simulink model "DinamicaCinematicaControleAtitude"  (R2024a)
settings: Solver=FixedStepAuto  StartTime=0.0  StopTime=tf  FixedStep=step_modelo  RelTol=1e-3
undefined symbols (not defined in the file or in its folder): giro, giro_bias, giro_ruido, Ixx, Iyy, Izz, omega1_rel_ini, omega2_rel_ini, omega3_rel_ini, phi_i, psi_i, theta_i
libraries: dspsrcs4 x3, matrix_library x2, aerolibutil x1
settings Model: Creator=rodri  LastModifiedBy=rodri
settings DataIOCC: SaveOutput=off  SaveTime=off
settings RTWCC: GPUComputeCapability=3.5

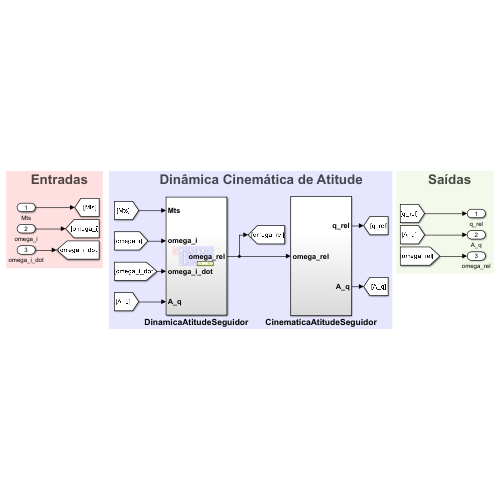
[thumbnail: Simulink's stored preview of the top-level diagram]
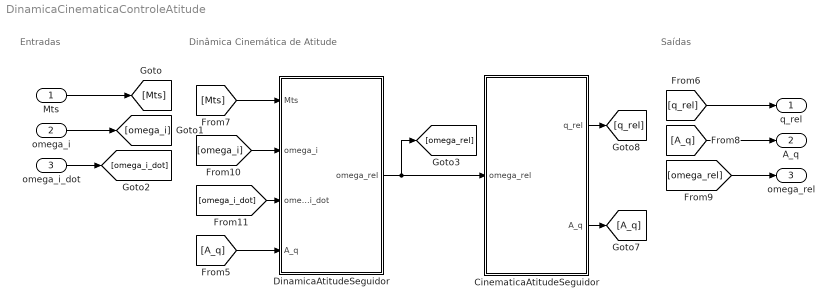
== system DinamicaCinematicaControleAtitude ==
  note: Dinâmica Cinemática de Atitude
  note: Entradas
  note: Saídas
  Mts : Inport  OutDataTypeStr=double  PortDimensions=[3,1]
  omega_i : Inport  Port=2  OutDataTypeStr=double
  omega_i_dot : Inport  Port=3  OutDataTypeStr=double  PortDimensions=[3,1]
  CinematicaAtitudeSeguidor : Subsystem
  DinamicaAtitudeSeguidor : Subsystem
  q_rel : Outport
  A_q : Outport  Port=2  PortDimensions=[3,3]
  omega_rel : Outport  Port=3
  wires:
  DinamicaAtitudeSeguidor/1(omega_rel) -> [omega_rel], CinematicaAtitudeSeguidor/1(omega_rel)
  CinematicaAtitudeSeguidor/2(A_q) -> [A_q]
  CinematicaAtitudeSeguidor/1(q_rel) -> [q_rel]
  omega_i/1 -> [omega_i]
  omega_i_dot/1 -> [omega_i_dot]
  [A_q] -> DinamicaAtitudeSeguidor/4(A_q)
  [Mts] -> DinamicaAtitudeSeguidor/1(Mts)
  [omega_i] -> DinamicaAtitudeSeguidor/2(omega_i)
  [omega_i_dot] -> DinamicaAtitudeSeguidor/3(omega_i_dot)
  [q_rel] -> q_rel/1
  [A_q] -> A_q/1
  [omega_rel] -> omega_rel/1
  Mts/1 -> [Mts]

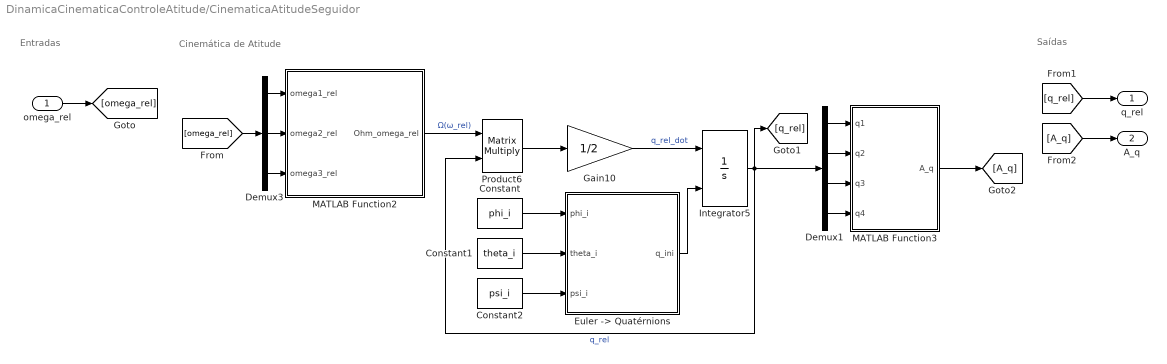
== system DinamicaCinematicaControleAtitude/CinematicaAtitudeSeguidor ==
  note: Cinemática de Atitude
  note: Entradas
  note: Saídas
  omega_rel : Inport
  Constant : Constant  Value=phi_i  SampleTime=-1
  Constant1 : Constant  Value=theta_i  SampleTime=-1
  Constant2 : Constant  Value=psi_i  SampleTime=-1
  Demux1 : Demux
  Demux3 : Demux  Outputs=3
  "Euler -> Quatérnions" : MATLAB Function  TreatAsAtomicUnit=on
  Gain10 : Gain  Gain=1/2
  Integrator5 : Integrator  InitialConditionSource=external  InitialCondition=[1; 0; 0; 0]
  MATLAB Function2 : MATLAB Function  TreatAsAtomicUnit=on
  MATLAB Function3 : MATLAB Function  TreatAsAtomicUnit=on
  Product6 : Product  Multiplication=Matrix(*)
  q_rel : Outport
  A_q : Outport  Port=2  PortDimensions=[3,3]
  wires:
  "Euler -> Quatérnions"/1(q_ini) -> Integrator5/2
  Demux1/2 -> MATLAB Function3/2(q2)
  Demux3/1 -> MATLAB Function2/1(omega1_rel)
  MATLAB Function2/1(Ohm_omega_rel) -> Product6/1  "Ω(ω_rel)"
  Demux1/4 -> MATLAB Function3/4(q4)
  Demux3/3 -> MATLAB Function2/3(omega3_rel)
  Demux3/2 -> MATLAB Function2/2(omega2_rel)
  Integrator5/1 -> Product6/2, Demux1/1, [q_rel]  "q_rel"
  Demux1/3 -> MATLAB Function3/3(q3)
  Gain10/1 -> Integrator5/1  "q_rel_dot"
  Demux1/1 -> MATLAB Function3/1(q1)
  Product6/1 -> Gain10/1
  [omega_rel] -> Demux3/1
  omega_rel/1 -> [omega_rel]
  [q_rel] -> q_rel/1
  [A_q] -> A_q/1
  MATLAB Function3/1(A_q) -> [A_q]
  Constant/1 -> "Euler -> Quatérnions"/1(phi_i)
  Constant1/1 -> "Euler -> Quatérnions"/2(theta_i)
  Constant2/1 -> "Euler -> Quatérnions"/3(psi_i)

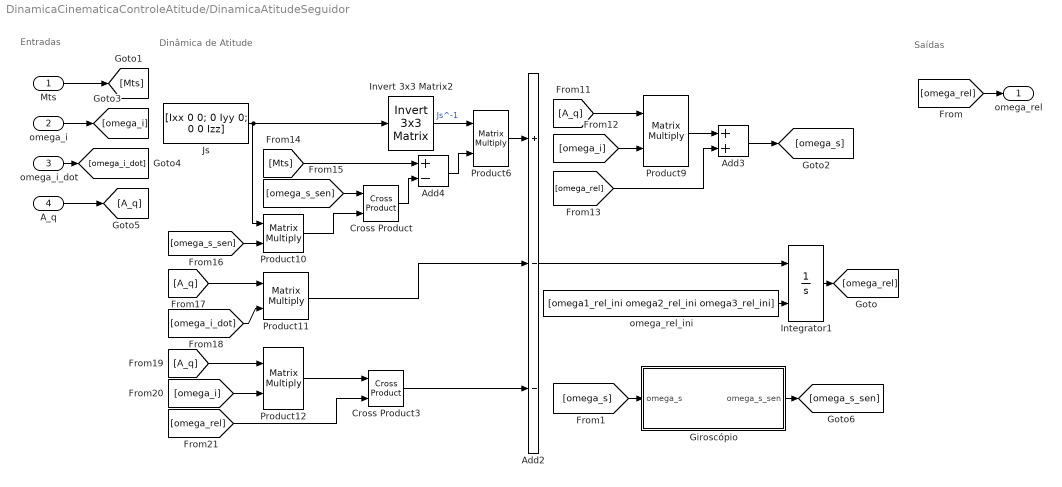
== system DinamicaCinematicaControleAtitude/DinamicaAtitudeSeguidor ==
  note: Dinâmica de Atitude
  note: Saídas
  note: Entradas
  Mts : Inport
  omega_i : Inport  Port=2
  omega_i_dot : Inport  Port=3
  A_q : Inport  Port=4
  Add2 : Sum  Inputs=+--
  Add3 : Sum
  Add4 : Sum  Inputs=+-
  Cross Product : matrix_library/Cross Product
  Cross Product3 : matrix_library/Cross Product
  Giroscópio : Subsystem
  Integrator1 : Integrator  InitialConditionSource=external  InitialCondition=[0; 0; 0]
  Invert 3x3 Matrix2 : aerolibutil/Invert  3x3 Matrix
  Js : Constant  Value=[Ixx 0 0; 0 Iyy 0; 0 0 Izz]
  Product{6,9..12} (5 alike) : Product  Multiplication=Matrix(*)
  omega_rel_ini : Constant  Value=[omega1_rel_ini omega2_rel_ini omega3_rel_ini]
  omega_rel : Outport
  wires:
  Integrator1/1 -> [omega_rel]
  Add2/1 -> Integrator1/1
  Invert 3x3 Matrix2/1 -> Product6/1  "Js^-1"
  omega_rel_ini/1 -> Integrator1/2
  [A_q] -> Product9/1
  [omega_i] -> Product9/2
  Product9/1 -> Add3/1
  [omega_rel] -> Add3/2
  Add3/1 -> [omega_s]
  [Mts] -> Add4/1
  Cross Product/1 -> Add4/2
  [omega_s_sen] -> Cross Product/1
  Js/1 -> Product10/1, Invert 3x3 Matrix2/1
  [omega_s_sen] -> Product10/2
  Product10/1 -> Cross Product/2
  Add4/1 -> Product6/2
  Product6/1 -> Add2/1
  [A_q] -> Product11/1
  [omega_i_dot] -> Product11/2
  Product11/1 -> Add2/2
  [A_q] -> Product12/1
  [omega_i] -> Product12/2
  Product12/1 -> Cross Product3/1
  [omega_rel] -> Cross Product3/2
  Cross Product3/1 -> Add2/3
  omega_i/1 -> [omega_i]
  A_q/1 -> [A_q]
  [omega_rel] -> omega_rel/1
  Mts/1 -> [Mts]
  omega_i_dot/1 -> [omega_i_dot]
  [omega_s] -> Giroscópio/1(omega_s)
  Giroscópio/1(omega_s_sen) -> [omega_s_sen]

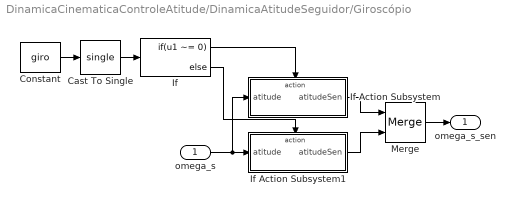
== system DinamicaCinematicaControleAtitude/DinamicaAtitudeSeguidor/Giroscópio ==
  omega_s : Inport
  Cast To Single : DataTypeConversion  OutDataTypeStr=single  SaturateOnIntegerOverflow=off  RndMeth=Floor
  Constant : Constant  Value=giro
  If : If  IfExpression=u1 ~= 0
  If Action Subsystem : Subsystem  TreatAsAtomicUnit=on
  If Action Subsystem1 : Subsystem  TreatAsAtomicUnit=on
  Merge : Merge
  omega_s_sen : Outport
  wires:
  Cast To Single/1 -> If/1
  If/2 -> If Action Subsystem1/Action
  If Action Subsystem/1(atitudeSen) -> Merge/1
  If/1 -> If Action Subsystem/Action
  Merge/1 -> omega_s_sen/1
  Constant/1 -> Cast To Single/1
  If Action Subsystem1/1(atitudeSen) -> Merge/2
  omega_s/1 -> If Action Subsystem/1(atitude), If Action Subsystem1/1(atitude)

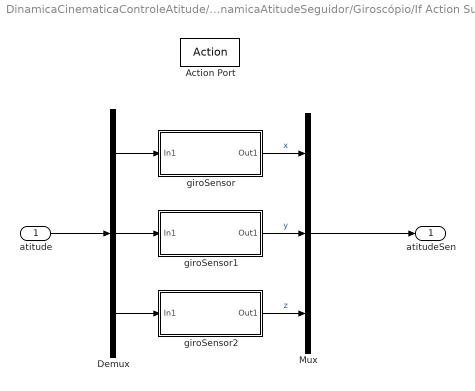
== system DinamicaCinematicaControleAtitude/DinamicaAtitudeSeguidor/Giroscópio/If Action Subsystem ==
  atitude : Inport
  Action Port : ActionPort  ActionPortLabel=if(u1 ~= 0)
  Demux : Demux  Outputs=3
  Mux : Mux  Inputs=3
  giroSensor : Subsystem
  giroSensor1 : Subsystem
  giroSensor2 : Subsystem
  atitudeSen : Outport
  wires:
  Demux/3 -> giroSensor2/1(In1)
  Demux/2 -> giroSensor1/1(In1)
  Demux/1 -> giroSensor/1(In1)
  atitude/1 -> Demux/1
  giroSensor/1(Out1) -> Mux/1  "x"
  giroSensor1/1(Out1) -> Mux/2  "y"
  giroSensor2/1(Out1) -> Mux/3  "z"
  Mux/1 -> atitudeSen/1

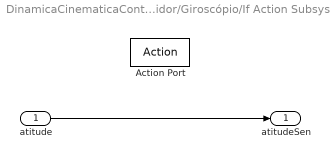
== system DinamicaCinematicaControleAtitude/DinamicaAtitudeSeguidor/Giroscópio/If Action Subsystem1 ==
  atitude : Inport
  Action Port : ActionPort  ActionPortLabel=else
  atitudeSen : Outport
  wires:
  atitude/1 -> atitudeSen/1

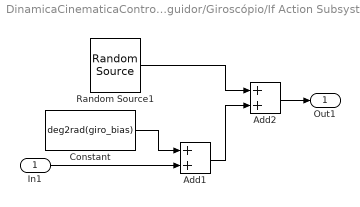
== system DinamicaCinematicaControleAtitude/DinamicaAtitudeSeguidor/Giroscópio/If Action Subsystem/giroSensor ==
  In1 : Inport
  Add1 : Sum
  Add2 : Sum
  Constant : Constant  Value=deg2rad(giro_bias)
  Random Source1 : dspsrcs4/Random Source  SrcType=Uniform  MinVal=-deg2rad(giro_ruido)  MaxVal=deg2rad(giro_ruido)  MeanVal=0  VarVal=1  RepMode=Not repeatable  rawSeed=1  IsInherit=off  SampTime=step_modelo  SampFrame=1  OutComplex=Real  DataType=double  SimulateUsing=Code generation
  Out1 : Outport
  wires:
  Random Source1/1 -> Add2/1
  In1/1 -> Add1/2
  Constant/1 -> Add1/1
  Add1/1 -> Add2/2
  Add2/1 -> Out1/1

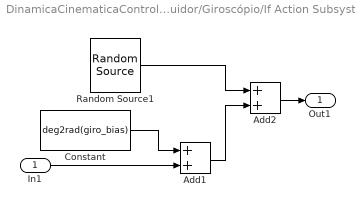
== system DinamicaCinematicaControleAtitude/DinamicaAtitudeSeguidor/Giroscópio/If Action Subsystem/giroSensor1 ==
  In1 : Inport
  Add1 : Sum
  Add2 : Sum
  Constant : Constant  Value=deg2rad(giro_bias)
  Random Source1 : dspsrcs4/Random Source  SrcType=Uniform  MinVal=-deg2rad(giro_ruido)  MaxVal=deg2rad(giro_ruido)  MeanVal=0  VarVal=1  RepMode=Not repeatable  rawSeed=1  IsInherit=off  SampTime=step_modelo  SampFrame=1  OutComplex=Real  DataType=double  SimulateUsing=Code generation
  Out1 : Outport
  wires:
  Random Source1/1 -> Add2/1
  Add2/1 -> Out1/1
  In1/1 -> Add1/2
  Constant/1 -> Add1/1
  Add1/1 -> Add2/2

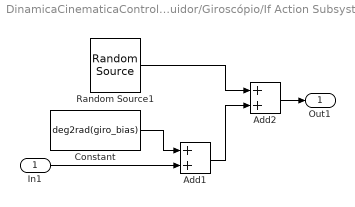
== system DinamicaCinematicaControleAtitude/DinamicaAtitudeSeguidor/Giroscópio/If Action Subsystem/giroSensor2 ==
  In1 : Inport
  Add1 : Sum
  Add2 : Sum
  Constant : Constant  Value=deg2rad(giro_bias)
  Random Source1 : dspsrcs4/Random Source  SrcType=Uniform  MinVal=-deg2rad(giro_ruido)  MaxVal=deg2rad(giro_ruido)  MeanVal=0  VarVal=1  RepMode=Not repeatable  rawSeed=1  IsInherit=off  SampTime=step_modelo  SampFrame=1  OutComplex=Real  DataType=double  SimulateUsing=Code generation
  Out1 : Outport
  wires:
  Random Source1/1 -> Add2/1
  Add2/1 -> Out1/1
  In1/1 -> Add1/2
  Constant/1 -> Add1/1
  Add1/1 -> Add2/2

== matlab function DinamicaCinematicaControleAtitude/CinematicaAtitudeSeguidor/MATLAB Function2 ==
  data: omega1_rel input; Ohm_omega_rel output; omega2_rel input; omega3_rel input
function Ohm_omega_rel  = fcn(omega1_rel,omega2_rel,omega3_rel)

Ohm_omega_rel = [0 omega3_rel -omega2_rel omega1_rel
    -omega3_rel 0 omega1_rel omega2_rel
    omega2_rel -omega1_rel 0 omega3_rel
    -omega1_rel -omega2_rel -omega3_rel 0];

== matlab function DinamicaCinematicaControleAtitude/CinematicaAtitudeSeguidor/MATLAB Function3 ==
  data: q1 input; A_q output; q2 input; q3 input; q4 input
function A_q = fcn(q1,q2,q3,q4)

A_q_11 = q1^2-q2^2-q3^2+q4^2;
A_q_12 = 2*(q1*q2+q3*q4);
A_q_13 = 2*(q1*q3-q2*q4);
A_q_21 = 2*(q1*q2-q3*q4);
A_q_22 = -q1^2+q2^2-q3^2+q4^2;
A_q_23 = 2*(q2*q3+q1*q4);
A_q_31 = 2*(q1*q3+q2*q4);
A_q_32 = 2*(q2*q3-q1*q4);
A_q_33 = -q1^2-q2^2+q3^2+q4^2;

A_q = [A_q_11, A_q_12, A_q_13;
       A_q_21, A_q_22, A_q_23;
       A_q_31, A_q_32, A_q_33];

== matlab function DinamicaCinematicaControleAtitude/CinematicaAtitudeSeguidor/Euler -> Quatérnions ==
  data: phi_i input; q_ini output; theta_i input; psi_i input
function q_ini = fcn(phi_i,theta_i,psi_i)

q_ref = eul2quat([phi_i theta_i psi_i]);

q_ini = [q_ref(2),q_ref(3),q_ref(4),q_ref(1)]';
